simulink model "NoC_4x4x3"  (R2015a)
settings: Solver=ode45  StartTime=0.0  StopTime=10.0  RelTol=1e-3
undefined symbols (not defined in the file or in its folder): des, SELECT
undefined symbols (not defined in the file): MAX, MIN, T
libraries: simulink x48
(part 10 of 12)

== system NoC_4x4x3/LayerDown/Sitch3DXYZ8/RouteXYZ ==
  Attribute Function : Subsystem  LoadFcn=des.afb.attributefunction_support(gcb,'LoadFcn');  StartFcn=des.afb.attributefunction_support(gcb,'StartFcn');  mask(Attribute Function){OutputNamePrefix=out_}
      mask prompts: OutputNamePrefix "Prefix name"
      settings: CopyFcn=des.afb.attributefunction_support(gcb,'CopyFcn');  OpenFcn=des.afb.attributefunction_support(gcb,'OpenFcn');  ErrorFcn=des.afb.error_redirect
      mask Help: slhelp(gcbh)
      mask Display: image(des_iconLoad('attribFunction.jpg'),'center');
  Set Attribute : SetAttribute  AttributeName=IME_X|IME_Y|IME_Z  AttributeFrom=Dialog|Dialog|Dialog  AttributeValue=ME_X|ME_Y|ME_Z  AttributeTreatAsVector=1|1|1  EvaluatedAttributeValue={ ME_X;ME_Y;ME_Z}
  Input : PMIOPort  Port=1  Side=Left
  Output : PMIOPort  Port=2  Side=Right
  connections:
  Input/RConn1 -- Set Attribute/LConn1
  Output/RConn1 -- Attribute Function/RConn1
  Set Attribute/RConn1 -- Attribute Function/LConn1

== system NoC_4x4x3/LayerDown/Sitch3DXYZ9/RouteXYZ ==
  Attribute Function : Subsystem  LoadFcn=des.afb.attributefunction_support(gcb,'LoadFcn');  StartFcn=des.afb.attributefunction_support(gcb,'StartFcn');  mask(Attribute Function){OutputNamePrefix=out_}
      mask prompts: OutputNamePrefix "Prefix name"
      settings: CopyFcn=des.afb.attributefunction_support(gcb,'CopyFcn');  OpenFcn=des.afb.attributefunction_support(gcb,'OpenFcn');  ErrorFcn=des.afb.error_redirect
      mask Help: slhelp(gcbh)
      mask Display: image(des_iconLoad('attribFunction.jpg'),'center');
  Set Attribute : SetAttribute  AttributeName=IME_X|IME_Y|IME_Z  AttributeFrom=Dialog|Dialog|Dialog  AttributeValue=ME_X|ME_Y|ME_Z  AttributeTreatAsVector=1|1|1  EvaluatedAttributeValue={ ME_X;ME_Y;ME_Z}
  Input : PMIOPort  Port=1  Side=Left
  Output : PMIOPort  Port=2  Side=Right
  connections:
  Set Attribute/RConn1 -- Attribute Function/LConn1
  Output/RConn1 -- Attribute Function/RConn1
  Input/RConn1 -- Set Attribute/LConn1

== system NoC_4x4x3/LayerUp/PE00/Create Generator Selection Variable ==
  function : TriggerPort  TriggerType=function-call
  Repeating Sequence Stair : simulink/Sources/Repeating Sequence Stair  OutValues=[0 1].'  tsamp=-1  OutMin=[]  OutMax=[]  OutDataTypeStr=float('double')  OutputDataTypeScalingMode=Specify via dialog  OutDataType=float('double')  ConRadixGroup=Best Precision: Vector-wise  OutScaling=2^-12
  Out1 : Outport
  wires:
  Repeating Sequence Stair/1 -> Out1/1

== system NoC_4x4x3/LayerUp/PE01/Create Generator Selection Variable ==
  function : TriggerPort  TriggerType=function-call
  Repeating Sequence Stair : simulink/Sources/Repeating Sequence Stair  OutValues=[0 1].'  tsamp=-1  OutMin=[]  OutMax=[]  OutDataTypeStr=float('double')  OutputDataTypeScalingMode=Specify via dialog  OutDataType=float('double')  ConRadixGroup=Best Precision: Vector-wise  OutScaling=2^-12
  Out1 : Outport
  wires:
  Repeating Sequence Stair/1 -> Out1/1

== system NoC_4x4x3/LayerUp/PE02/Create Generator Selection Variable ==
  function : TriggerPort  TriggerType=function-call
  Repeating Sequence Stair : simulink/Sources/Repeating Sequence Stair  OutValues=[0 1].'  tsamp=-1  OutMin=[]  OutMax=[]  OutDataTypeStr=float('double')  OutputDataTypeScalingMode=Specify via dialog  OutDataType=float('double')  ConRadixGroup=Best Precision: Vector-wise  OutScaling=2^-12
  Out1 : Outport
  wires:
  Repeating Sequence Stair/1 -> Out1/1

== system NoC_4x4x3/LayerUp/PE03/Create Generator Selection Variable ==
  function : TriggerPort  TriggerType=function-call
  Repeating Sequence Stair : simulink/Sources/Repeating Sequence Stair  OutValues=[0 1].'  tsamp=-1  OutMin=[]  OutMax=[]  OutDataTypeStr=float('double')  OutputDataTypeScalingMode=Specify via dialog  OutDataType=float('double')  ConRadixGroup=Best Precision: Vector-wise  OutScaling=2^-12
  Out1 : Outport
  wires:
  Repeating Sequence Stair/1 -> Out1/1

== system NoC_4x4x3/LayerUp/PE10/Create Generator Selection Variable ==
  function : TriggerPort  TriggerType=function-call
  Repeating Sequence Stair : simulink/Sources/Repeating Sequence Stair  OutValues=[0 1].'  tsamp=-1  OutMin=[]  OutMax=[]  OutDataTypeStr=float('double')  OutputDataTypeScalingMode=Specify via dialog  OutDataType=float('double')  ConRadixGroup=Best Precision: Vector-wise  OutScaling=2^-12
  Out1 : Outport
  wires:
  Repeating Sequence Stair/1 -> Out1/1

== system NoC_4x4x3/LayerUp/PE11/Create Generator Selection Variable ==
  function : TriggerPort  TriggerType=function-call
  Repeating Sequence Stair : simulink/Sources/Repeating Sequence Stair  OutValues=[0 1].'  tsamp=-1  OutMin=[]  OutMax=[]  OutDataTypeStr=float('double')  OutputDataTypeScalingMode=Specify via dialog  OutDataType=float('double')  ConRadixGroup=Best Precision: Vector-wise  OutScaling=2^-12
  Out1 : Outport
  wires:
  Repeating Sequence Stair/1 -> Out1/1

== system NoC_4x4x3/LayerUp/PE12/Create Generator Selection Variable ==
  function : TriggerPort  TriggerType=function-call
  Repeating Sequence Stair : simulink/Sources/Repeating Sequence Stair  OutValues=[0 1].'  tsamp=-1  OutMin=[]  OutMax=[]  OutDataTypeStr=float('double')  OutputDataTypeScalingMode=Specify via dialog  OutDataType=float('double')  ConRadixGroup=Best Precision: Vector-wise  OutScaling=2^-12
  Out1 : Outport
  wires:
  Repeating Sequence Stair/1 -> Out1/1

== system NoC_4x4x3/LayerUp/PE13/Create Generator Selection Variable ==
  function : TriggerPort  TriggerType=function-call
  Repeating Sequence Stair : simulink/Sources/Repeating Sequence Stair  OutValues=[0 1].'  tsamp=-1  OutMin=[]  OutMax=[]  OutDataTypeStr=float('double')  OutputDataTypeScalingMode=Specify via dialog  OutDataType=float('double')  ConRadixGroup=Best Precision: Vector-wise  OutScaling=2^-12
  Out1 : Outport
  wires:
  Repeating Sequence Stair/1 -> Out1/1

== system NoC_4x4x3/LayerUp/PE20/Create Generator Selection Variable ==
  function : TriggerPort  TriggerType=function-call
  Repeating Sequence Stair : simulink/Sources/Repeating Sequence Stair  OutValues=[0 1].'  tsamp=-1  OutMin=[]  OutMax=[]  OutDataTypeStr=float('double')  OutputDataTypeScalingMode=Specify via dialog  OutDataType=float('double')  ConRadixGroup=Best Precision: Vector-wise  OutScaling=2^-12
  Out1 : Outport
  wires:
  Repeating Sequence Stair/1 -> Out1/1

== system NoC_4x4x3/LayerUp/PE21/Create Generator Selection Variable ==
  function : TriggerPort  TriggerType=function-call
  Repeating Sequence Stair : simulink/Sources/Repeating Sequence Stair  OutValues=[0 1].'  tsamp=-1  OutMin=[]  OutMax=[]  OutDataTypeStr=float('double')  OutputDataTypeScalingMode=Specify via dialog  OutDataType=float('double')  ConRadixGroup=Best Precision: Vector-wise  OutScaling=2^-12
  Out1 : Outport
  wires:
  Repeating Sequence Stair/1 -> Out1/1

== system NoC_4x4x3/LayerUp/PE22/Create Generator Selection Variable ==
  function : TriggerPort  TriggerType=function-call
  Repeating Sequence Stair : simulink/Sources/Repeating Sequence Stair  OutValues=[0 1].'  tsamp=-1  OutMin=[]  OutMax=[]  OutDataTypeStr=float('double')  OutputDataTypeScalingMode=Specify via dialog  OutDataType=float('double')  ConRadixGroup=Best Precision: Vector-wise  OutScaling=2^-12
  Out1 : Outport
  wires:
  Repeating Sequence Stair/1 -> Out1/1

== system NoC_4x4x3/LayerUp/PE23/Create Generator Selection Variable ==
  function : TriggerPort  TriggerType=function-call
  Repeating Sequence Stair : simulink/Sources/Repeating Sequence Stair  OutValues=[0 1].'  tsamp=-1  OutMin=[]  OutMax=[]  OutDataTypeStr=float('double')  OutputDataTypeScalingMode=Specify via dialog  OutDataType=float('double')  ConRadixGroup=Best Precision: Vector-wise  OutScaling=2^-12
  Out1 : Outport
  wires:
  Repeating Sequence Stair/1 -> Out1/1

== system NoC_4x4x3/LayerUp/PE30/Create Generator Selection Variable ==
  function : TriggerPort  TriggerType=function-call
  Repeating Sequence Stair : simulink/Sources/Repeating Sequence Stair  OutValues=[0 1].'  tsamp=-1  OutMin=[]  OutMax=[]  OutDataTypeStr=float('double')  OutputDataTypeScalingMode=Specify via dialog  OutDataType=float('double')  ConRadixGroup=Best Precision: Vector-wise  OutScaling=2^-12
  Out1 : Outport
  wires:
  Repeating Sequence Stair/1 -> Out1/1

== system NoC_4x4x3/LayerUp/PE31/Create Generator Selection Variable ==
  function : TriggerPort  TriggerType=function-call
  Repeating Sequence Stair : simulink/Sources/Repeating Sequence Stair  OutValues=[0 1].'  tsamp=-1  OutMin=[]  OutMax=[]  OutDataTypeStr=float('double')  OutputDataTypeScalingMode=Specify via dialog  OutDataType=float('double')  ConRadixGroup=Best Precision: Vector-wise  OutScaling=2^-12
  Out1 : Outport
  wires:
  Repeating Sequence Stair/1 -> Out1/1

== system NoC_4x4x3/LayerUp/PE32/Create Generator Selection Variable ==
  function : TriggerPort  TriggerType=function-call
  Repeating Sequence Stair : simulink/Sources/Repeating Sequence Stair  OutValues=[0 1].'  tsamp=-1  OutMin=[]  OutMax=[]  OutDataTypeStr=float('double')  OutputDataTypeScalingMode=Specify via dialog  OutDataType=float('double')  ConRadixGroup=Best Precision: Vector-wise  OutScaling=2^-12
  Out1 : Outport
  wires:
  Repeating Sequence Stair/1 -> Out1/1

== system NoC_4x4x3/LayerUp/PE33/Create Generator Selection Variable ==
  function : TriggerPort  TriggerType=function-call
  Repeating Sequence Stair : simulink/Sources/Repeating Sequence Stair  OutValues=[0 1].'  tsamp=-1  OutMin=[]  OutMax=[]  OutDataTypeStr=float('double')  OutputDataTypeScalingMode=Specify via dialog  OutDataType=float('double')  ConRadixGroup=Best Precision: Vector-wise  OutScaling=2^-12
  Out1 : Outport
  wires:
  Repeating Sequence Stair/1 -> Out1/1

== system NoC_4x4x3/LayerUp/Sitch3DXYZ/RouteXYZ ==
  Attribute Function : Subsystem  LoadFcn=des.afb.attributefunction_support(gcb,'LoadFcn');  StartFcn=des.afb.attributefunction_support(gcb,'StartFcn');  mask(Attribute Function){OutputNamePrefix=out_}
      mask prompts: OutputNamePrefix "Prefix name"
      settings: CopyFcn=des.afb.attributefunction_support(gcb,'CopyFcn');  OpenFcn=des.afb.attributefunction_support(gcb,'OpenFcn');  ErrorFcn=des.afb.error_redirect
      mask Help: slhelp(gcbh)
      mask Display: image(des_iconLoad('attribFunction.jpg'),'center');
  Set Attribute : SetAttribute  AttributeName=IME_X|IME_Y|IME_Z  AttributeFrom=Dialog|Dialog|Dialog  AttributeValue=ME_X|ME_Y|ME_Z  AttributeTreatAsVector=1|1|1  EvaluatedAttributeValue={ ME_X;ME_Y;ME_Z}
  Input : PMIOPort  Port=1  Side=Left
  Output : PMIOPort  Port=2  Side=Right
  connections:
  Input/RConn1 -- Set Attribute/LConn1
  Output/RConn1 -- Attribute Function/RConn1
  Set Attribute/RConn1 -- Attribute Function/LConn1

== system NoC_4x4x3/LayerUp/Sitch3DXYZ1/RouteXYZ ==
  Attribute Function : Subsystem  LoadFcn=des.afb.attributefunction_support(gcb,'LoadFcn');  StartFcn=des.afb.attributefunction_support(gcb,'StartFcn');  mask(Attribute Function){OutputNamePrefix=out_}
      mask prompts: OutputNamePrefix "Prefix name"
      settings: CopyFcn=des.afb.attributefunction_support(gcb,'CopyFcn');  OpenFcn=des.afb.attributefunction_support(gcb,'OpenFcn');  ErrorFcn=des.afb.error_redirect
      mask Help: slhelp(gcbh)
      mask Display: image(des_iconLoad('attribFunction.jpg'),'center');
  Set Attribute : SetAttribute  AttributeName=IME_X|IME_Y|IME_Z  AttributeFrom=Dialog|Dialog|Dialog  AttributeValue=ME_X|ME_Y|ME_Z  AttributeTreatAsVector=1|1|1  EvaluatedAttributeValue={ ME_X;ME_Y;ME_Z}
  Input : PMIOPort  Port=1  Side=Left
  Output : PMIOPort  Port=2  Side=Right
  connections:
  Set Attribute/RConn1 -- Attribute Function/LConn1
  Output/RConn1 -- Attribute Function/RConn1
  Input/RConn1 -- Set Attribute/LConn1

== system NoC_4x4x3/LayerUp/Sitch3DXYZ10/RouteXYZ ==
  Attribute Function : Subsystem  LoadFcn=des.afb.attributefunction_support(gcb,'LoadFcn');  StartFcn=des.afb.attributefunction_support(gcb,'StartFcn');  mask(Attribute Function){OutputNamePrefix=out_}
      mask prompts: OutputNamePrefix "Prefix name"
      settings: CopyFcn=des.afb.attributefunction_support(gcb,'CopyFcn');  OpenFcn=des.afb.attributefunction_support(gcb,'OpenFcn');  ErrorFcn=des.afb.error_redirect
      mask Help: slhelp(gcbh)
      mask Display: image(des_iconLoad('attribFunction.jpg'),'center');
  Set Attribute : SetAttribute  AttributeName=IME_X|IME_Y|IME_Z  AttributeFrom=Dialog|Dialog|Dialog  AttributeValue=ME_X|ME_Y|ME_Z  AttributeTreatAsVector=1|1|1  EvaluatedAttributeValue={ ME_X;ME_Y;ME_Z}
  Input : PMIOPort  Port=1  Side=Left
  Output : PMIOPort  Port=2  Side=Right
  connections:
  Input/RConn1 -- Set Attribute/LConn1
  Output/RConn1 -- Attribute Function/RConn1
  Set Attribute/RConn1 -- Attribute Function/LConn1

== system NoC_4x4x3/LayerUp/Sitch3DXYZ11/RouteXYZ ==
  Attribute Function : Subsystem  LoadFcn=des.afb.attributefunction_support(gcb,'LoadFcn');  StartFcn=des.afb.attributefunction_support(gcb,'StartFcn');  mask(Attribute Function){OutputNamePrefix=out_}
      mask prompts: OutputNamePrefix "Prefix name"
      settings: CopyFcn=des.afb.attributefunction_support(gcb,'CopyFcn');  OpenFcn=des.afb.attributefunction_support(gcb,'OpenFcn');  ErrorFcn=des.afb.error_redirect
      mask Help: slhelp(gcbh)
      mask Display: image(des_iconLoad('attribFunction.jpg'),'center');
  Set Attribute : SetAttribute  AttributeName=IME_X|IME_Y|IME_Z  AttributeFrom=Dialog|Dialog|Dialog  AttributeValue=ME_X|ME_Y|ME_Z  AttributeTreatAsVector=1|1|1  EvaluatedAttributeValue={ ME_X;ME_Y;ME_Z}
  Input : PMIOPort  Port=1  Side=Left
  Output : PMIOPort  Port=2  Side=Right
  connections:
  Set Attribute/RConn1 -- Attribute Function/LConn1
  Output/RConn1 -- Attribute Function/RConn1
  Input/RConn1 -- Set Attribute/LConn1

== system NoC_4x4x3/LayerUp/Sitch3DXYZ12/RouteXYZ ==
  Attribute Function : Subsystem  LoadFcn=des.afb.attributefunction_support(gcb,'LoadFcn');  StartFcn=des.afb.attributefunction_support(gcb,'StartFcn');  mask(Attribute Function){OutputNamePrefix=out_}
      mask prompts: OutputNamePrefix "Prefix name"
      settings: CopyFcn=des.afb.attributefunction_support(gcb,'CopyFcn');  OpenFcn=des.afb.attributefunction_support(gcb,'OpenFcn');  ErrorFcn=des.afb.error_redirect
      mask Help: slhelp(gcbh)
      mask Display: image(des_iconLoad('attribFunction.jpg'),'center');
  Set Attribute : SetAttribute  AttributeName=IME_X|IME_Y|IME_Z  AttributeFrom=Dialog|Dialog|Dialog  AttributeValue=ME_X|ME_Y|ME_Z  AttributeTreatAsVector=1|1|1  EvaluatedAttributeValue={ ME_X;ME_Y;ME_Z}
  Input : PMIOPort  Port=1  Side=Left
  Output : PMIOPort  Port=2  Side=Right
  connections:
  Set Attribute/RConn1 -- Attribute Function/LConn1
  Output/RConn1 -- Attribute Function/RConn1
  Input/RConn1 -- Set Attribute/LConn1

== system NoC_4x4x3/LayerUp/Sitch3DXYZ13/RouteXYZ ==
  Attribute Function : Subsystem  LoadFcn=des.afb.attributefunction_support(gcb,'LoadFcn');  StartFcn=des.afb.attributefunction_support(gcb,'StartFcn');  mask(Attribute Function){OutputNamePrefix=out_}
      mask prompts: OutputNamePrefix "Prefix name"
      settings: CopyFcn=des.afb.attributefunction_support(gcb,'CopyFcn');  OpenFcn=des.afb.attributefunction_support(gcb,'OpenFcn');  ErrorFcn=des.afb.error_redirect
      mask Help: slhelp(gcbh)
      mask Display: image(des_iconLoad('attribFunction.jpg'),'center');
  Set Attribute : SetAttribute  AttributeName=IME_X|IME_Y|IME_Z  AttributeFrom=Dialog|Dialog|Dialog  AttributeValue=ME_X|ME_Y|ME_Z  AttributeTreatAsVector=1|1|1  EvaluatedAttributeValue={ ME_X;ME_Y;ME_Z}
  Input : PMIOPort  Port=1  Side=Left
  Output : PMIOPort  Port=2  Side=Right
  connections:
  Input/RConn1 -- Set Attribute/LConn1
  Output/RConn1 -- Attribute Function/RConn1
  Set Attribute/RConn1 -- Attribute Function/LConn1

== system NoC_4x4x3/LayerUp/Sitch3DXYZ14/RouteXYZ ==
  Attribute Function : Subsystem  LoadFcn=des.afb.attributefunction_support(gcb,'LoadFcn');  StartFcn=des.afb.attributefunction_support(gcb,'StartFcn');  mask(Attribute Function){OutputNamePrefix=out_}
      mask prompts: OutputNamePrefix "Prefix name"
      settings: CopyFcn=des.afb.attributefunction_support(gcb,'CopyFcn');  OpenFcn=des.afb.attributefunction_support(gcb,'OpenFcn');  ErrorFcn=des.afb.error_redirect
      mask Help: slhelp(gcbh)
      mask Display: image(des_iconLoad('attribFunction.jpg'),'center');
  Set Attribute : SetAttribute  AttributeName=IME_X|IME_Y|IME_Z  AttributeFrom=Dialog|Dialog|Dialog  AttributeValue=ME_X|ME_Y|ME_Z  AttributeTreatAsVector=1|1|1  EvaluatedAttributeValue={ ME_X;ME_Y;ME_Z}
  Input : PMIOPort  Port=1  Side=Left
  Output : PMIOPort  Port=2  Side=Right
  connections:
  Set Attribute/RConn1 -- Attribute Function/LConn1
  Output/RConn1 -- Attribute Function/RConn1
  Input/RConn1 -- Set Attribute/LConn1

== system NoC_4x4x3/LayerUp/Sitch3DXYZ15/RouteXYZ ==
  Attribute Function : Subsystem  LoadFcn=des.afb.attributefunction_support(gcb,'LoadFcn');  StartFcn=des.afb.attributefunction_support(gcb,'StartFcn');  mask(Attribute Function){OutputNamePrefix=out_}
      mask prompts: OutputNamePrefix "Prefix name"
      settings: CopyFcn=des.afb.attributefunction_support(gcb,'CopyFcn');  OpenFcn=des.afb.attributefunction_support(gcb,'OpenFcn');  ErrorFcn=des.afb.error_redirect
      mask Help: slhelp(gcbh)
      mask Display: image(des_iconLoad('attribFunction.jpg'),'center');
  Set Attribute : SetAttribute  AttributeName=IME_X|IME_Y|IME_Z  AttributeFrom=Dialog|Dialog|Dialog  AttributeValue=ME_X|ME_Y|ME_Z  AttributeTreatAsVector=1|1|1  EvaluatedAttributeValue={ ME_X;ME_Y;ME_Z}
  Input : PMIOPort  Port=1  Side=Left
  Output : PMIOPort  Port=2  Side=Right
  connections:
  Input/RConn1 -- Set Attribute/LConn1
  Output/RConn1 -- Attribute Function/RConn1
  Set Attribute/RConn1 -- Attribute Function/LConn1

== system NoC_4x4x3/LayerUp/Sitch3DXYZ2/RouteXYZ ==
  Attribute Function : Subsystem  LoadFcn=des.afb.attributefunction_support(gcb,'LoadFcn');  StartFcn=des.afb.attributefunction_support(gcb,'StartFcn');  mask(Attribute Function){OutputNamePrefix=out_}
      mask prompts: OutputNamePrefix "Prefix name"
      settings: CopyFcn=des.afb.attributefunction_support(gcb,'CopyFcn');  OpenFcn=des.afb.attributefunction_support(gcb,'OpenFcn');  ErrorFcn=des.afb.error_redirect
      mask Help: slhelp(gcbh)
      mask Display: image(des_iconLoad('attribFunction.jpg'),'center');
  Set Attribute : SetAttribute  AttributeName=IME_X|IME_Y|IME_Z  AttributeFrom=Dialog|Dialog|Dialog  AttributeValue=ME_X|ME_Y|ME_Z  AttributeTreatAsVector=1|1|1  EvaluatedAttributeValue={ ME_X;ME_Y;ME_Z}
  Input : PMIOPort  Port=1  Side=Left
  Output : PMIOPort  Port=2  Side=Right
  connections:
  Input/RConn1 -- Set Attribute/LConn1
  Output/RConn1 -- Attribute Function/RConn1
  Set Attribute/RConn1 -- Attribute Function/LConn1

== system NoC_4x4x3/LayerUp/Sitch3DXYZ3/RouteXYZ ==
  Attribute Function : Subsystem  LoadFcn=des.afb.attributefunction_support(gcb,'LoadFcn');  StartFcn=des.afb.attributefunction_support(gcb,'StartFcn');  mask(Attribute Function){OutputNamePrefix=out_}
      mask prompts: OutputNamePrefix "Prefix name"
      settings: CopyFcn=des.afb.attributefunction_support(gcb,'CopyFcn');  OpenFcn=des.afb.attributefunction_support(gcb,'OpenFcn');  ErrorFcn=des.afb.error_redirect
      mask Help: slhelp(gcbh)
      mask Display: image(des_iconLoad('attribFunction.jpg'),'center');
  Set Attribute : SetAttribute  AttributeName=IME_X|IME_Y|IME_Z  AttributeFrom=Dialog|Dialog|Dialog  AttributeValue=ME_X|ME_Y|ME_Z  AttributeTreatAsVector=1|1|1  EvaluatedAttributeValue={ ME_X;ME_Y;ME_Z}
  Input : PMIOPort  Port=1  Side=Left
  Output : PMIOPort  Port=2  Side=Right
  connections:
  Set Attribute/RConn1 -- Attribute Function/LConn1
  Output/RConn1 -- Attribute Function/RConn1
  Input/RConn1 -- Set Attribute/LConn1

== system NoC_4x4x3/LayerUp/Sitch3DXYZ4/RouteXYZ ==
  Attribute Function : Subsystem  LoadFcn=des.afb.attributefunction_support(gcb,'LoadFcn');  StartFcn=des.afb.attributefunction_support(gcb,'StartFcn');  mask(Attribute Function){OutputNamePrefix=out_}
      mask prompts: OutputNamePrefix "Prefix name"
      settings: CopyFcn=des.afb.attributefunction_support(gcb,'CopyFcn');  OpenFcn=des.afb.attributefunction_support(gcb,'OpenFcn');  ErrorFcn=des.afb.error_redirect
      mask Help: slhelp(gcbh)
      mask Display: image(des_iconLoad('attribFunction.jpg'),'center');
  Set Attribute : SetAttribute  AttributeName=IME_X|IME_Y|IME_Z  AttributeFrom=Dialog|Dialog|Dialog  AttributeValue=ME_X|ME_Y|ME_Z  AttributeTreatAsVector=1|1|1  EvaluatedAttributeValue={ ME_X;ME_Y;ME_Z}
  Input : PMIOPort  Port=1  Side=Left
  Output : PMIOPort  Port=2  Side=Right
  connections:
  Set Attribute/RConn1 -- Attribute Function/LConn1
  Output/RConn1 -- Attribute Function/RConn1
  Input/RConn1 -- Set Attribute/LConn1

== system NoC_4x4x3/LayerUp/Sitch3DXYZ5/RouteXYZ ==
  Attribute Function : Subsystem  LoadFcn=des.afb.attributefunction_support(gcb,'LoadFcn');  StartFcn=des.afb.attributefunction_support(gcb,'StartFcn');  mask(Attribute Function){OutputNamePrefix=out_}
      mask prompts: OutputNamePrefix "Prefix name"
      settings: CopyFcn=des.afb.attributefunction_support(gcb,'CopyFcn');  OpenFcn=des.afb.attributefunction_support(gcb,'OpenFcn');  ErrorFcn=des.afb.error_redirect
      mask Help: slhelp(gcbh)
      mask Display: image(des_iconLoad('attribFunction.jpg'),'center');
  Set Attribute : SetAttribute  AttributeName=IME_X|IME_Y|IME_Z  AttributeFrom=Dialog|Dialog|Dialog  AttributeValue=ME_X|ME_Y|ME_Z  AttributeTreatAsVector=1|1|1  EvaluatedAttributeValue={ ME_X;ME_Y;ME_Z}
  Input : PMIOPort  Port=1  Side=Left
  Output : PMIOPort  Port=2  Side=Right
  connections:
  Input/RConn1 -- Set Attribute/LConn1
  Output/RConn1 -- Attribute Function/RConn1
  Set Attribute/RConn1 -- Attribute Function/LConn1

== system NoC_4x4x3/LayerUp/Sitch3DXYZ6/RouteXYZ ==
  Attribute Function : Subsystem  LoadFcn=des.afb.attributefunction_support(gcb,'LoadFcn');  StartFcn=des.afb.attributefunction_support(gcb,'StartFcn');  mask(Attribute Function){OutputNamePrefix=out_}
      mask prompts: OutputNamePrefix "Prefix name"
      settings: CopyFcn=des.afb.attributefunction_support(gcb,'CopyFcn');  OpenFcn=des.afb.attributefunction_support(gcb,'OpenFcn');  ErrorFcn=des.afb.error_redirect
      mask Help: slhelp(gcbh)
      mask Display: image(des_iconLoad('attribFunction.jpg'),'center');
  Set Attribute : SetAttribute  AttributeName=IME_X|IME_Y|IME_Z  AttributeFrom=Dialog|Dialog|Dialog  AttributeValue=ME_X|ME_Y|ME_Z  AttributeTreatAsVector=1|1|1  EvaluatedAttributeValue={ ME_X;ME_Y;ME_Z}
  Input : PMIOPort  Port=1  Side=Left
  Output : PMIOPort  Port=2  Side=Right
  connections:
  Set Attribute/RConn1 -- Attribute Function/LConn1
  Output/RConn1 -- Attribute Function/RConn1
  Input/RConn1 -- Set Attribute/LConn1

== system NoC_4x4x3/LayerUp/Sitch3DXYZ7/RouteXYZ ==
  Attribute Function : Subsystem  LoadFcn=des.afb.attributefunction_support(gcb,'LoadFcn');  StartFcn=des.afb.attributefunction_support(gcb,'StartFcn');  mask(Attribute Function){OutputNamePrefix=out_}
      mask prompts: OutputNamePrefix "Prefix name"
      settings: CopyFcn=des.afb.attributefunction_support(gcb,'CopyFcn');  OpenFcn=des.afb.attributefunction_support(gcb,'OpenFcn');  ErrorFcn=des.afb.error_redirect
      mask Help: slhelp(gcbh)
      mask Display: image(des_iconLoad('attribFunction.jpg'),'center');
  Set Attribute : SetAttribute  AttributeName=IME_X|IME_Y|IME_Z  AttributeFrom=Dialog|Dialog|Dialog  AttributeValue=ME_X|ME_Y|ME_Z  AttributeTreatAsVector=1|1|1  EvaluatedAttributeValue={ ME_X;ME_Y;ME_Z}
  Input : PMIOPort  Port=1  Side=Left
  Output : PMIOPort  Port=2  Side=Right
  connections:
  Input/RConn1 -- Set Attribute/LConn1
  Output/RConn1 -- Attribute Function/RConn1
  Set Attribute/RConn1 -- Attribute Function/LConn1

== system NoC_4x4x3/LayerUp/Sitch3DXYZ8/RouteXYZ ==
  Attribute Function : Subsystem  LoadFcn=des.afb.attributefunction_support(gcb,'LoadFcn');  StartFcn=des.afb.attributefunction_support(gcb,'StartFcn');  mask(Attribute Function){OutputNamePrefix=out_}
      mask prompts: OutputNamePrefix "Prefix name"
      settings: CopyFcn=des.afb.attributefunction_support(gcb,'CopyFcn');  OpenFcn=des.afb.attributefunction_support(gcb,'OpenFcn');  ErrorFcn=des.afb.error_redirect
      mask Help: slhelp(gcbh)
      mask Display: image(des_iconLoad('attribFunction.jpg'),'center');
  Set Attribute : SetAttribute  AttributeName=IME_X|IME_Y|IME_Z  AttributeFrom=Dialog|Dialog|Dialog  AttributeValue=ME_X|ME_Y|ME_Z  AttributeTreatAsVector=1|1|1  EvaluatedAttributeValue={ ME_X;ME_Y;ME_Z}
  Input : PMIOPort  Port=1  Side=Left
  Output : PMIOPort  Port=2  Side=Right
  connections:
  Input/RConn1 -- Set Attribute/LConn1
  Output/RConn1 -- Attribute Function/RConn1
  Set Attribute/RConn1 -- Attribute Function/LConn1

== system NoC_4x4x3/LayerUp/Sitch3DXYZ9/RouteXYZ ==
  Attribute Function : Subsystem  LoadFcn=des.afb.attributefunction_support(gcb,'LoadFcn');  StartFcn=des.afb.attributefunction_support(gcb,'StartFcn');  mask(Attribute Function){OutputNamePrefix=out_}
      mask prompts: OutputNamePrefix "Prefix name"
      settings: CopyFcn=des.afb.attributefunction_support(gcb,'CopyFcn');  OpenFcn=des.afb.attributefunction_support(gcb,'OpenFcn');  ErrorFcn=des.afb.error_redirect
      mask Help: slhelp(gcbh)
      mask Display: image(des_iconLoad('attribFunction.jpg'),'center');
  Set Attribute : SetAttribute  AttributeName=IME_X|IME_Y|IME_Z  AttributeFrom=Dialog|Dialog|Dialog  AttributeValue=ME_X|ME_Y|ME_Z  AttributeTreatAsVector=1|1|1  EvaluatedAttributeValue={ ME_X;ME_Y;ME_Z}
  Input : PMIOPort  Port=1  Side=Left
  Output : PMIOPort  Port=2  Side=Right
  connections:
  Set Attribute/RConn1 -- Attribute Function/LConn1
  Output/RConn1 -- Attribute Function/RConn1
  Input/RConn1 -- Set Attribute/LConn1

== system NoC_4x4x3/Layer/Sitch3DXYZ/RouteXYZ/Attribute Function ==
  MATLAB Function : MATLAB Function  TreatAsAtomicUnit=on
  __DMLF__EDE2FCE__ : EntityDepartureFunctionCallGenerator  TimingFunctionCallF1=Before entity departure  IsInsideAFB=on
  __DMLF__GA__ : GetAttribute  AttributeName=DST_X|DST_Y|DST_Z|IME_X|IME_Y|IME_Z  AttributeMissing=Error|Error|Error|Error|Error|Error  AttributeDefaultValue=1|1|1|1|1|1  AttributeTreatAsVector=1|1|1|1|1|1  AttributeSendTiming=Before entity departure|Before entity departure|Before entity departure|Before entity departure|Before entity departure|Before entity departure  EvaluatedDefaultAttributeValue={ [];[];[];[];[];[]}  IsInsideAFB=on
      settings: OutputPortMap=o1,o2,o3,o4,o5,o6
  __DMLF__SA__ : SetAttribute  AttributeName=RT  AttributeFrom=Signal port  EvaluatedAttributeValue={ []}  IsInsideAFB=on
  IN : PMIOPort  Port=1  Side=Left
  OUT : PMIOPort  Port=2  Side=Right
  wires:
  __DMLF__EDE2FCE__/1 -> MATLAB Function/Trigger
  __DMLF__GA__/1 -> MATLAB Function/1(DST_X)
  __DMLF__GA__/2 -> MATLAB Function/2(DST_Y)
  __DMLF__GA__/3 -> MATLAB Function/3(DST_Z)
  __DMLF__GA__/4 -> MATLAB Function/4(IME_X)
  __DMLF__GA__/5 -> MATLAB Function/5(IME_Y)
  __DMLF__GA__/6 -> MATLAB Function/6(IME_Z)
  MATLAB Function/1(out_RT) -> __DMLF__SA__/1
  connections:
  __DMLF__SA__/LConn1 -- __DMLF__EDE2FCE__/RConn1
  __DMLF__GA__/RConn1 -- __DMLF__EDE2FCE__/LConn1
  IN/RConn1 -- __DMLF__GA__/LConn1
  __DMLF__SA__/RConn1 -- OUT/RConn1

== system NoC_4x4x3/Layer/Sitch3DXYZ1/RouteXYZ/Attribute Function ==
  MATLAB Function : MATLAB Function  TreatAsAtomicUnit=on
  __DMLF__EDE2FCE__ : EntityDepartureFunctionCallGenerator  TimingFunctionCallF1=Before entity departure  IsInsideAFB=on
  __DMLF__GA__ : GetAttribute  AttributeName=DST_X|DST_Y|DST_Z|IME_X|IME_Y|IME_Z  AttributeMissing=Error|Error|Error|Error|Error|Error  AttributeDefaultValue=1|1|1|1|1|1  AttributeTreatAsVector=1|1|1|1|1|1  AttributeSendTiming=Before entity departure|Before entity departure|Before entity departure|Before entity departure|Before entity departure|Before entity departure  EvaluatedDefaultAttributeValue={ [];[];[];[];[];[]}  IsInsideAFB=on
      settings: OutputPortMap=o1,o2,o3,o4,o5,o6
  __DMLF__SA__ : SetAttribute  AttributeName=RT  AttributeFrom=Signal port  EvaluatedAttributeValue={ []}  IsInsideAFB=on
  IN : PMIOPort  Port=1  Side=Left
  OUT : PMIOPort  Port=2  Side=Right
  wires:
  __DMLF__EDE2FCE__/1 -> MATLAB Function/Trigger
  __DMLF__GA__/1 -> MATLAB Function/1(DST_X)
  __DMLF__GA__/2 -> MATLAB Function/2(DST_Y)
  __DMLF__GA__/3 -> MATLAB Function/3(DST_Z)
  __DMLF__GA__/4 -> MATLAB Function/4(IME_X)
  __DMLF__GA__/5 -> MATLAB Function/5(IME_Y)
  __DMLF__GA__/6 -> MATLAB Function/6(IME_Z)
  MATLAB Function/1(out_RT) -> __DMLF__SA__/1
  connections:
  __DMLF__SA__/RConn1 -- OUT/RConn1
  IN/RConn1 -- __DMLF__GA__/LConn1
  __DMLF__GA__/RConn1 -- __DMLF__EDE2FCE__/LConn1
  __DMLF__SA__/LConn1 -- __DMLF__EDE2FCE__/RConn1

== system NoC_4x4x3/Layer/Sitch3DXYZ10/RouteXYZ/Attribute Function ==
  MATLAB Function : MATLAB Function  TreatAsAtomicUnit=on
  __DMLF__EDE2FCE__ : EntityDepartureFunctionCallGenerator  TimingFunctionCallF1=Before entity departure  IsInsideAFB=on
  __DMLF__GA__ : GetAttribute  AttributeName=DST_X|DST_Y|DST_Z|IME_X|IME_Y|IME_Z  AttributeMissing=Error|Error|Error|Error|Error|Error  AttributeDefaultValue=1|1|1|1|1|1  AttributeTreatAsVector=1|1|1|1|1|1  AttributeSendTiming=Before entity departure|Before entity departure|Before entity departure|Before entity departure|Before entity departure|Before entity departure  EvaluatedDefaultAttributeValue={ [];[];[];[];[];[]}  IsInsideAFB=on
      settings: OutputPortMap=o1,o2,o3,o4,o5,o6
  __DMLF__SA__ : SetAttribute  AttributeName=RT  AttributeFrom=Signal port  EvaluatedAttributeValue={ []}  IsInsideAFB=on
  IN : PMIOPort  Port=1  Side=Left
  OUT : PMIOPort  Port=2  Side=Right
  wires:
  __DMLF__EDE2FCE__/1 -> MATLAB Function/Trigger
  __DMLF__GA__/1 -> MATLAB Function/1(DST_X)
  __DMLF__GA__/2 -> MATLAB Function/2(DST_Y)
  __DMLF__GA__/3 -> MATLAB Function/3(DST_Z)
  __DMLF__GA__/4 -> MATLAB Function/4(IME_X)
  __DMLF__GA__/5 -> MATLAB Function/5(IME_Y)
  __DMLF__GA__/6 -> MATLAB Function/6(IME_Z)
  MATLAB Function/1(out_RT) -> __DMLF__SA__/1
  connections:
  __DMLF__SA__/LConn1 -- __DMLF__EDE2FCE__/RConn1
  __DMLF__GA__/RConn1 -- __DMLF__EDE2FCE__/LConn1
  IN/RConn1 -- __DMLF__GA__/LConn1
  __DMLF__SA__/RConn1 -- OUT/RConn1

== system NoC_4x4x3/Layer/Sitch3DXYZ11/RouteXYZ/Attribute Function ==
  MATLAB Function : MATLAB Function  TreatAsAtomicUnit=on
  __DMLF__EDE2FCE__ : EntityDepartureFunctionCallGenerator  TimingFunctionCallF1=Before entity departure  IsInsideAFB=on
  __DMLF__GA__ : GetAttribute  AttributeName=DST_X|DST_Y|DST_Z|IME_X|IME_Y|IME_Z  AttributeMissing=Error|Error|Error|Error|Error|Error  AttributeDefaultValue=1|1|1|1|1|1  AttributeTreatAsVector=1|1|1|1|1|1  AttributeSendTiming=Before entity departure|Before entity departure|Before entity departure|Before entity departure|Before entity departure|Before entity departure  EvaluatedDefaultAttributeValue={ [];[];[];[];[];[]}  IsInsideAFB=on
      settings: OutputPortMap=o1,o2,o3,o4,o5,o6
  __DMLF__SA__ : SetAttribute  AttributeName=RT  AttributeFrom=Signal port  EvaluatedAttributeValue={ []}  IsInsideAFB=on
  IN : PMIOPort  Port=1  Side=Left
  OUT : PMIOPort  Port=2  Side=Right
  wires:
  __DMLF__EDE2FCE__/1 -> MATLAB Function/Trigger
  __DMLF__GA__/1 -> MATLAB Function/1(DST_X)
  __DMLF__GA__/2 -> MATLAB Function/2(DST_Y)
  __DMLF__GA__/3 -> MATLAB Function/3(DST_Z)
  __DMLF__GA__/4 -> MATLAB Function/4(IME_X)
  __DMLF__GA__/5 -> MATLAB Function/5(IME_Y)
  __DMLF__GA__/6 -> MATLAB Function/6(IME_Z)
  MATLAB Function/1(out_RT) -> __DMLF__SA__/1
  connections:
  __DMLF__SA__/RConn1 -- OUT/RConn1
  IN/RConn1 -- __DMLF__GA__/LConn1
  __DMLF__GA__/RConn1 -- __DMLF__EDE2FCE__/LConn1
  __DMLF__SA__/LConn1 -- __DMLF__EDE2FCE__/RConn1

== system NoC_4x4x3/Layer/Sitch3DXYZ12/RouteXYZ/Attribute Function ==
  MATLAB Function : MATLAB Function  TreatAsAtomicUnit=on
  __DMLF__EDE2FCE__ : EntityDepartureFunctionCallGenerator  TimingFunctionCallF1=Before entity departure  IsInsideAFB=on
  __DMLF__GA__ : GetAttribute  AttributeName=DST_X|DST_Y|DST_Z|IME_X|IME_Y|IME_Z  AttributeMissing=Error|Error|Error|Error|Error|Error  AttributeDefaultValue=1|1|1|1|1|1  AttributeTreatAsVector=1|1|1|1|1|1  AttributeSendTiming=Before entity departure|Before entity departure|Before entity departure|Before entity departure|Before entity departure|Before entity departure  EvaluatedDefaultAttributeValue={ [];[];[];[];[];[]}  IsInsideAFB=on
      settings: OutputPortMap=o1,o2,o3,o4,o5,o6
  __DMLF__SA__ : SetAttribute  AttributeName=RT  AttributeFrom=Signal port  EvaluatedAttributeValue={ []}  IsInsideAFB=on
  IN : PMIOPort  Port=1  Side=Left
  OUT : PMIOPort  Port=2  Side=Right
  wires:
  __DMLF__EDE2FCE__/1 -> MATLAB Function/Trigger
  __DMLF__GA__/1 -> MATLAB Function/1(DST_X)
  __DMLF__GA__/2 -> MATLAB Function/2(DST_Y)
  __DMLF__GA__/3 -> MATLAB Function/3(DST_Z)
  __DMLF__GA__/4 -> MATLAB Function/4(IME_X)
  __DMLF__GA__/5 -> MATLAB Function/5(IME_Y)
  __DMLF__GA__/6 -> MATLAB Function/6(IME_Z)
  MATLAB Function/1(out_RT) -> __DMLF__SA__/1
  connections:
  __DMLF__SA__/RConn1 -- OUT/RConn1
  IN/RConn1 -- __DMLF__GA__/LConn1
  __DMLF__GA__/RConn1 -- __DMLF__EDE2FCE__/LConn1
  __DMLF__SA__/LConn1 -- __DMLF__EDE2FCE__/RConn1

== system NoC_4x4x3/Layer/Sitch3DXYZ13/RouteXYZ/Attribute Function ==
  MATLAB Function : MATLAB Function  TreatAsAtomicUnit=on
  __DMLF__EDE2FCE__ : EntityDepartureFunctionCallGenerator  TimingFunctionCallF1=Before entity departure  IsInsideAFB=on
  __DMLF__GA__ : GetAttribute  AttributeName=DST_X|DST_Y|DST_Z|IME_X|IME_Y|IME_Z  AttributeMissing=Error|Error|Error|Error|Error|Error  AttributeDefaultValue=1|1|1|1|1|1  AttributeTreatAsVector=1|1|1|1|1|1  AttributeSendTiming=Before entity departure|Before entity departure|Before entity departure|Before entity departure|Before entity departure|Before entity departure  EvaluatedDefaultAttributeValue={ [];[];[];[];[];[]}  IsInsideAFB=on
      settings: OutputPortMap=o1,o2,o3,o4,o5,o6
  __DMLF__SA__ : SetAttribute  AttributeName=RT  AttributeFrom=Signal port  EvaluatedAttributeValue={ []}  IsInsideAFB=on
  IN : PMIOPort  Port=1  Side=Left
  OUT : PMIOPort  Port=2  Side=Right
  wires:
  __DMLF__EDE2FCE__/1 -> MATLAB Function/Trigger
  __DMLF__GA__/1 -> MATLAB Function/1(DST_X)
  __DMLF__GA__/2 -> MATLAB Function/2(DST_Y)
  __DMLF__GA__/3 -> MATLAB Function/3(DST_Z)
  __DMLF__GA__/4 -> MATLAB Function/4(IME_X)
  __DMLF__GA__/5 -> MATLAB Function/5(IME_Y)
  __DMLF__GA__/6 -> MATLAB Function/6(IME_Z)
  MATLAB Function/1(out_RT) -> __DMLF__SA__/1
  connections:
  __DMLF__SA__/LConn1 -- __DMLF__EDE2FCE__/RConn1
  __DMLF__GA__/RConn1 -- __DMLF__EDE2FCE__/LConn1
  IN/RConn1 -- __DMLF__GA__/LConn1
  __DMLF__SA__/RConn1 -- OUT/RConn1

== system NoC_4x4x3/Layer/Sitch3DXYZ14/RouteXYZ/Attribute Function ==
  MATLAB Function : MATLAB Function  TreatAsAtomicUnit=on
  __DMLF__EDE2FCE__ : EntityDepartureFunctionCallGenerator  TimingFunctionCallF1=Before entity departure  IsInsideAFB=on
  __DMLF__GA__ : GetAttribute  AttributeName=DST_X|DST_Y|DST_Z|IME_X|IME_Y|IME_Z  AttributeMissing=Error|Error|Error|Error|Error|Error  AttributeDefaultValue=1|1|1|1|1|1  AttributeTreatAsVector=1|1|1|1|1|1  AttributeSendTiming=Before entity departure|Before entity departure|Before entity departure|Before entity departure|Before entity departure|Before entity departure  EvaluatedDefaultAttributeValue={ [];[];[];[];[];[]}  IsInsideAFB=on
      settings: OutputPortMap=o1,o2,o3,o4,o5,o6
  __DMLF__SA__ : SetAttribute  AttributeName=RT  AttributeFrom=Signal port  EvaluatedAttributeValue={ []}  IsInsideAFB=on
  IN : PMIOPort  Port=1  Side=Left
  OUT : PMIOPort  Port=2  Side=Right
  wires:
  __DMLF__EDE2FCE__/1 -> MATLAB Function/Trigger
  __DMLF__GA__/1 -> MATLAB Function/1(DST_X)
  __DMLF__GA__/2 -> MATLAB Function/2(DST_Y)
  __DMLF__GA__/3 -> MATLAB Function/3(DST_Z)
  __DMLF__GA__/4 -> MATLAB Function/4(IME_X)
  __DMLF__GA__/5 -> MATLAB Function/5(IME_Y)
  __DMLF__GA__/6 -> MATLAB Function/6(IME_Z)
  MATLAB Function/1(out_RT) -> __DMLF__SA__/1
  connections:
  __DMLF__SA__/RConn1 -- OUT/RConn1
  IN/RConn1 -- __DMLF__GA__/LConn1
  __DMLF__GA__/RConn1 -- __DMLF__EDE2FCE__/LConn1
  __DMLF__SA__/LConn1 -- __DMLF__EDE2FCE__/RConn1

== system NoC_4x4x3/Layer/Sitch3DXYZ15/RouteXYZ/Attribute Function ==
  MATLAB Function : MATLAB Function  TreatAsAtomicUnit=on
  __DMLF__EDE2FCE__ : EntityDepartureFunctionCallGenerator  TimingFunctionCallF1=Before entity departure  IsInsideAFB=on
  __DMLF__GA__ : GetAttribute  AttributeName=DST_X|DST_Y|DST_Z|IME_X|IME_Y|IME_Z  AttributeMissing=Error|Error|Error|Error|Error|Error  AttributeDefaultValue=1|1|1|1|1|1  AttributeTreatAsVector=1|1|1|1|1|1  AttributeSendTiming=Before entity departure|Before entity departure|Before entity departure|Before entity departure|Before entity departure|Before entity departure  EvaluatedDefaultAttributeValue={ [];[];[];[];[];[]}  IsInsideAFB=on
      settings: OutputPortMap=o1,o2,o3,o4,o5,o6
  __DMLF__SA__ : SetAttribute  AttributeName=RT  AttributeFrom=Signal port  EvaluatedAttributeValue={ []}  IsInsideAFB=on
  IN : PMIOPort  Port=1  Side=Left
  OUT : PMIOPort  Port=2  Side=Right
  wires:
  __DMLF__EDE2FCE__/1 -> MATLAB Function/Trigger
  __DMLF__GA__/1 -> MATLAB Function/1(DST_X)
  __DMLF__GA__/2 -> MATLAB Function/2(DST_Y)
  __DMLF__GA__/3 -> MATLAB Function/3(DST_Z)
  __DMLF__GA__/4 -> MATLAB Function/4(IME_X)
  __DMLF__GA__/5 -> MATLAB Function/5(IME_Y)
  __DMLF__GA__/6 -> MATLAB Function/6(IME_Z)
  MATLAB Function/1(out_RT) -> __DMLF__SA__/1
  connections:
  __DMLF__SA__/LConn1 -- __DMLF__EDE2FCE__/RConn1
  __DMLF__GA__/RConn1 -- __DMLF__EDE2FCE__/LConn1
  IN/RConn1 -- __DMLF__GA__/LConn1
  __DMLF__SA__/RConn1 -- OUT/RConn1

== system NoC_4x4x3/Layer/Sitch3DXYZ2/RouteXYZ/Attribute Function ==
  MATLAB Function : MATLAB Function  TreatAsAtomicUnit=on
  __DMLF__EDE2FCE__ : EntityDepartureFunctionCallGenerator  TimingFunctionCallF1=Before entity departure  IsInsideAFB=on
  __DMLF__GA__ : GetAttribute  AttributeName=DST_X|DST_Y|DST_Z|IME_X|IME_Y|IME_Z  AttributeMissing=Error|Error|Error|Error|Error|Error  AttributeDefaultValue=1|1|1|1|1|1  AttributeTreatAsVector=1|1|1|1|1|1  AttributeSendTiming=Before entity departure|Before entity departure|Before entity departure|Before entity departure|Before entity departure|Before entity departure  EvaluatedDefaultAttributeValue={ [];[];[];[];[];[]}  IsInsideAFB=on
      settings: OutputPortMap=o1,o2,o3,o4,o5,o6
  __DMLF__SA__ : SetAttribute  AttributeName=RT  AttributeFrom=Signal port  EvaluatedAttributeValue={ []}  IsInsideAFB=on
  IN : PMIOPort  Port=1  Side=Left
  OUT : PMIOPort  Port=2  Side=Right
  wires:
  __DMLF__EDE2FCE__/1 -> MATLAB Function/Trigger
  __DMLF__GA__/1 -> MATLAB Function/1(DST_X)
  __DMLF__GA__/2 -> MATLAB Function/2(DST_Y)
  __DMLF__GA__/3 -> MATLAB Function/3(DST_Z)
  __DMLF__GA__/4 -> MATLAB Function/4(IME_X)
  __DMLF__GA__/5 -> MATLAB Function/5(IME_Y)
  __DMLF__GA__/6 -> MATLAB Function/6(IME_Z)
  MATLAB Function/1(out_RT) -> __DMLF__SA__/1
  connections:
  __DMLF__SA__/LConn1 -- __DMLF__EDE2FCE__/RConn1
  __DMLF__GA__/RConn1 -- __DMLF__EDE2FCE__/LConn1
  IN/RConn1 -- __DMLF__GA__/LConn1
  __DMLF__SA__/RConn1 -- OUT/RConn1

== system NoC_4x4x3/Layer/Sitch3DXYZ3/RouteXYZ/Attribute Function ==
  MATLAB Function : MATLAB Function  TreatAsAtomicUnit=on
  __DMLF__EDE2FCE__ : EntityDepartureFunctionCallGenerator  TimingFunctionCallF1=Before entity departure  IsInsideAFB=on
  __DMLF__GA__ : GetAttribute  AttributeName=DST_X|DST_Y|DST_Z|IME_X|IME_Y|IME_Z  AttributeMissing=Error|Error|Error|Error|Error|Error  AttributeDefaultValue=1|1|1|1|1|1  AttributeTreatAsVector=1|1|1|1|1|1  AttributeSendTiming=Before entity departure|Before entity departure|Before entity departure|Before entity departure|Before entity departure|Before entity departure  EvaluatedDefaultAttributeValue={ [];[];[];[];[];[]}  IsInsideAFB=on
      settings: OutputPortMap=o1,o2,o3,o4,o5,o6
  __DMLF__SA__ : SetAttribute  AttributeName=RT  AttributeFrom=Signal port  EvaluatedAttributeValue={ []}  IsInsideAFB=on
  IN : PMIOPort  Port=1  Side=Left
  OUT : PMIOPort  Port=2  Side=Right
  wires:
  __DMLF__EDE2FCE__/1 -> MATLAB Function/Trigger
  __DMLF__GA__/1 -> MATLAB Function/1(DST_X)
  __DMLF__GA__/2 -> MATLAB Function/2(DST_Y)
  __DMLF__GA__/3 -> MATLAB Function/3(DST_Z)
  __DMLF__GA__/4 -> MATLAB Function/4(IME_X)
  __DMLF__GA__/5 -> MATLAB Function/5(IME_Y)
  __DMLF__GA__/6 -> MATLAB Function/6(IME_Z)
  MATLAB Function/1(out_RT) -> __DMLF__SA__/1
  connections:
  __DMLF__SA__/RConn1 -- OUT/RConn1
  IN/RConn1 -- __DMLF__GA__/LConn1
  __DMLF__GA__/RConn1 -- __DMLF__EDE2FCE__/LConn1
  __DMLF__SA__/LConn1 -- __DMLF__EDE2FCE__/RConn1

== system NoC_4x4x3/Layer/Sitch3DXYZ4/RouteXYZ/Attribute Function ==
  MATLAB Function : MATLAB Function  TreatAsAtomicUnit=on
  __DMLF__EDE2FCE__ : EntityDepartureFunctionCallGenerator  TimingFunctionCallF1=Before entity departure  IsInsideAFB=on
  __DMLF__GA__ : GetAttribute  AttributeName=DST_X|DST_Y|DST_Z|IME_X|IME_Y|IME_Z  AttributeMissing=Error|Error|Error|Error|Error|Error  AttributeDefaultValue=1|1|1|1|1|1  AttributeTreatAsVector=1|1|1|1|1|1  AttributeSendTiming=Before entity departure|Before entity departure|Before entity departure|Before entity departure|Before entity departure|Before entity departure  EvaluatedDefaultAttributeValue={ [];[];[];[];[];[]}  IsInsideAFB=on
      settings: OutputPortMap=o1,o2,o3,o4,o5,o6
  __DMLF__SA__ : SetAttribute  AttributeName=RT  AttributeFrom=Signal port  EvaluatedAttributeValue={ []}  IsInsideAFB=on
  IN : PMIOPort  Port=1  Side=Left
  OUT : PMIOPort  Port=2  Side=Right
  wires:
  __DMLF__EDE2FCE__/1 -> MATLAB Function/Trigger
  __DMLF__GA__/1 -> MATLAB Function/1(DST_X)
  __DMLF__GA__/2 -> MATLAB Function/2(DST_Y)
  __DMLF__GA__/3 -> MATLAB Function/3(DST_Z)
  __DMLF__GA__/4 -> MATLAB Function/4(IME_X)
  __DMLF__GA__/5 -> MATLAB Function/5(IME_Y)
  __DMLF__GA__/6 -> MATLAB Function/6(IME_Z)
  MATLAB Function/1(out_RT) -> __DMLF__SA__/1
  connections:
  __DMLF__SA__/RConn1 -- OUT/RConn1
  IN/RConn1 -- __DMLF__GA__/LConn1
  __DMLF__GA__/RConn1 -- __DMLF__EDE2FCE__/LConn1
  __DMLF__SA__/LConn1 -- __DMLF__EDE2FCE__/RConn1

== system NoC_4x4x3/Layer/Sitch3DXYZ5/RouteXYZ/Attribute Function ==
  MATLAB Function : MATLAB Function  TreatAsAtomicUnit=on
  __DMLF__EDE2FCE__ : EntityDepartureFunctionCallGenerator  TimingFunctionCallF1=Before entity departure  IsInsideAFB=on
  __DMLF__GA__ : GetAttribute  AttributeName=DST_X|DST_Y|DST_Z|IME_X|IME_Y|IME_Z  AttributeMissing=Error|Error|Error|Error|Error|Error  AttributeDefaultValue=1|1|1|1|1|1  AttributeTreatAsVector=1|1|1|1|1|1  AttributeSendTiming=Before entity departure|Before entity departure|Before entity departure|Before entity departure|Before entity departure|Before entity departure  EvaluatedDefaultAttributeValue={ [];[];[];[];[];[]}  IsInsideAFB=on
      settings: OutputPortMap=o1,o2,o3,o4,o5,o6
  __DMLF__SA__ : SetAttribute  AttributeName=RT  AttributeFrom=Signal port  EvaluatedAttributeValue={ []}  IsInsideAFB=on
  IN : PMIOPort  Port=1  Side=Left
  OUT : PMIOPort  Port=2  Side=Right
  wires:
  __DMLF__EDE2FCE__/1 -> MATLAB Function/Trigger
  __DMLF__GA__/1 -> MATLAB Function/1(DST_X)
  __DMLF__GA__/2 -> MATLAB Function/2(DST_Y)
  __DMLF__GA__/3 -> MATLAB Function/3(DST_Z)
  __DMLF__GA__/4 -> MATLAB Function/4(IME_X)
  __DMLF__GA__/5 -> MATLAB Function/5(IME_Y)
  __DMLF__GA__/6 -> MATLAB Function/6(IME_Z)
  MATLAB Function/1(out_RT) -> __DMLF__SA__/1
  connections:
  __DMLF__SA__/LConn1 -- __DMLF__EDE2FCE__/RConn1
  __DMLF__GA__/RConn1 -- __DMLF__EDE2FCE__/LConn1
  IN/RConn1 -- __DMLF__GA__/LConn1
  __DMLF__SA__/RConn1 -- OUT/RConn1

== system NoC_4x4x3/Layer/Sitch3DXYZ6/RouteXYZ/Attribute Function ==
  MATLAB Function : MATLAB Function  TreatAsAtomicUnit=on
  __DMLF__EDE2FCE__ : EntityDepartureFunctionCallGenerator  TimingFunctionCallF1=Before entity departure  IsInsideAFB=on
  __DMLF__GA__ : GetAttribute  AttributeName=DST_X|DST_Y|DST_Z|IME_X|IME_Y|IME_Z  AttributeMissing=Error|Error|Error|Error|Error|Error  AttributeDefaultValue=1|1|1|1|1|1  AttributeTreatAsVector=1|1|1|1|1|1  AttributeSendTiming=Before entity departure|Before entity departure|Before entity departure|Before entity departure|Before entity departure|Before entity departure  EvaluatedDefaultAttributeValue={ [];[];[];[];[];[]}  IsInsideAFB=on
      settings: OutputPortMap=o1,o2,o3,o4,o5,o6
  __DMLF__SA__ : SetAttribute  AttributeName=RT  AttributeFrom=Signal port  EvaluatedAttributeValue={ []}  IsInsideAFB=on
  IN : PMIOPort  Port=1  Side=Left
  OUT : PMIOPort  Port=2  Side=Right
  wires:
  __DMLF__EDE2FCE__/1 -> MATLAB Function/Trigger
  __DMLF__GA__/1 -> MATLAB Function/1(DST_X)
  __DMLF__GA__/2 -> MATLAB Function/2(DST_Y)
  __DMLF__GA__/3 -> MATLAB Function/3(DST_Z)
  __DMLF__GA__/4 -> MATLAB Function/4(IME_X)
  __DMLF__GA__/5 -> MATLAB Function/5(IME_Y)
  __DMLF__GA__/6 -> MATLAB Function/6(IME_Z)
  MATLAB Function/1(out_RT) -> __DMLF__SA__/1
  connections:
  __DMLF__SA__/RConn1 -- OUT/RConn1
  IN/RConn1 -- __DMLF__GA__/LConn1
  __DMLF__GA__/RConn1 -- __DMLF__EDE2FCE__/LConn1
  __DMLF__SA__/LConn1 -- __DMLF__EDE2FCE__/RConn1

== system NoC_4x4x3/Layer/Sitch3DXYZ7/RouteXYZ/Attribute Function ==
  MATLAB Function : MATLAB Function  TreatAsAtomicUnit=on
  __DMLF__EDE2FCE__ : EntityDepartureFunctionCallGenerator  TimingFunctionCallF1=Before entity departure  IsInsideAFB=on
  __DMLF__GA__ : GetAttribute  AttributeName=DST_X|DST_Y|DST_Z|IME_X|IME_Y|IME_Z  AttributeMissing=Error|Error|Error|Error|Error|Error  AttributeDefaultValue=1|1|1|1|1|1  AttributeTreatAsVector=1|1|1|1|1|1  AttributeSendTiming=Before entity departure|Before entity departure|Before entity departure|Before entity departure|Before entity departure|Before entity departure  EvaluatedDefaultAttributeValue={ [];[];[];[];[];[]}  IsInsideAFB=on
      settings: OutputPortMap=o1,o2,o3,o4,o5,o6
  __DMLF__SA__ : SetAttribute  AttributeName=RT  AttributeFrom=Signal port  EvaluatedAttributeValue={ []}  IsInsideAFB=on
  IN : PMIOPort  Port=1  Side=Left
  OUT : PMIOPort  Port=2  Side=Right
  wires:
  __DMLF__EDE2FCE__/1 -> MATLAB Function/Trigger
  __DMLF__GA__/1 -> MATLAB Function/1(DST_X)
  __DMLF__GA__/2 -> MATLAB Function/2(DST_Y)
  __DMLF__GA__/3 -> MATLAB Function/3(DST_Z)
  __DMLF__GA__/4 -> MATLAB Function/4(IME_X)
  __DMLF__GA__/5 -> MATLAB Function/5(IME_Y)
  __DMLF__GA__/6 -> MATLAB Function/6(IME_Z)
  MATLAB Function/1(out_RT) -> __DMLF__SA__/1
  connections:
  __DMLF__SA__/LConn1 -- __DMLF__EDE2FCE__/RConn1
  __DMLF__GA__/RConn1 -- __DMLF__EDE2FCE__/LConn1
  IN/RConn1 -- __DMLF__GA__/LConn1
  __DMLF__SA__/RConn1 -- OUT/RConn1

== system NoC_4x4x3/Layer/Sitch3DXYZ8/RouteXYZ/Attribute Function ==
  MATLAB Function : MATLAB Function  TreatAsAtomicUnit=on
  __DMLF__EDE2FCE__ : EntityDepartureFunctionCallGenerator  TimingFunctionCallF1=Before entity departure  IsInsideAFB=on
  __DMLF__GA__ : GetAttribute  AttributeName=DST_X|DST_Y|DST_Z|IME_X|IME_Y|IME_Z  AttributeMissing=Error|Error|Error|Error|Error|Error  AttributeDefaultValue=1|1|1|1|1|1  AttributeTreatAsVector=1|1|1|1|1|1  AttributeSendTiming=Before entity departure|Before entity departure|Before entity departure|Before entity departure|Before entity departure|Before entity departure  EvaluatedDefaultAttributeValue={ [];[];[];[];[];[]}  IsInsideAFB=on
      settings: OutputPortMap=o1,o2,o3,o4,o5,o6
  __DMLF__SA__ : SetAttribute  AttributeName=RT  AttributeFrom=Signal port  EvaluatedAttributeValue={ []}  IsInsideAFB=on
  IN : PMIOPort  Port=1  Side=Left
  OUT : PMIOPort  Port=2  Side=Right
  wires:
  __DMLF__EDE2FCE__/1 -> MATLAB Function/Trigger
  __DMLF__GA__/1 -> MATLAB Function/1(DST_X)
  __DMLF__GA__/2 -> MATLAB Function/2(DST_Y)
  __DMLF__GA__/3 -> MATLAB Function/3(DST_Z)
  __DMLF__GA__/4 -> MATLAB Function/4(IME_X)
  __DMLF__GA__/5 -> MATLAB Function/5(IME_Y)
  __DMLF__GA__/6 -> MATLAB Function/6(IME_Z)
  MATLAB Function/1(out_RT) -> __DMLF__SA__/1
  connections:
  __DMLF__SA__/LConn1 -- __DMLF__EDE2FCE__/RConn1
  __DMLF__GA__/RConn1 -- __DMLF__EDE2FCE__/LConn1
  IN/RConn1 -- __DMLF__GA__/LConn1
  __DMLF__SA__/RConn1 -- OUT/RConn1

== system NoC_4x4x3/Layer/Sitch3DXYZ9/RouteXYZ/Attribute Function ==
  MATLAB Function : MATLAB Function  TreatAsAtomicUnit=on
  __DMLF__EDE2FCE__ : EntityDepartureFunctionCallGenerator  TimingFunctionCallF1=Before entity departure  IsInsideAFB=on
  __DMLF__GA__ : GetAttribute  AttributeName=DST_X|DST_Y|DST_Z|IME_X|IME_Y|IME_Z  AttributeMissing=Error|Error|Error|Error|Error|Error  AttributeDefaultValue=1|1|1|1|1|1  AttributeTreatAsVector=1|1|1|1|1|1  AttributeSendTiming=Before entity departure|Before entity departure|Before entity departure|Before entity departure|Before entity departure|Before entity departure  EvaluatedDefaultAttributeValue={ [];[];[];[];[];[]}  IsInsideAFB=on
      settings: OutputPortMap=o1,o2,o3,o4,o5,o6
  __DMLF__SA__ : SetAttribute  AttributeName=RT  AttributeFrom=Signal port  EvaluatedAttributeValue={ []}  IsInsideAFB=on
  IN : PMIOPort  Port=1  Side=Left
  OUT : PMIOPort  Port=2  Side=Right
  wires:
  __DMLF__EDE2FCE__/1 -> MATLAB Function/Trigger
  __DMLF__GA__/1 -> MATLAB Function/1(DST_X)
  __DMLF__GA__/2 -> MATLAB Function/2(DST_Y)
  __DMLF__GA__/3 -> MATLAB Function/3(DST_Z)
  __DMLF__GA__/4 -> MATLAB Function/4(IME_X)
  __DMLF__GA__/5 -> MATLAB Function/5(IME_Y)
  __DMLF__GA__/6 -> MATLAB Function/6(IME_Z)
  MATLAB Function/1(out_RT) -> __DMLF__SA__/1
  connections:
  __DMLF__SA__/RConn1 -- OUT/RConn1
  IN/RConn1 -- __DMLF__GA__/LConn1
  __DMLF__GA__/RConn1 -- __DMLF__EDE2FCE__/LConn1
  __DMLF__SA__/LConn1 -- __DMLF__EDE2FCE__/RConn1
